simulink model "Lab2_Model"  (R2017a)
settings: Solver=VariableStepAuto  StartTime=0.0  StopTime=2  RelTol=1e-3
values from neighbouring files (symbols this model uses):
  C_D = c2d(C,0.005,'tustin')    [Lab2.m]    (also in Lab3.m = c2d(C,T,'tustin'))
  K1 = 0.66538    [Lab2.m]    (also in Lab3.m)
  Kp = 15    [Lab2.m]    (also in Lab3.m)
  p = 10.5    [Lab2.m]    (also in Lab3.m)
  T = 0.005    [Lab2.m]    (also in Lab3.m; Lab3calculations.m)
  tau = 0.030541    [Lab2.m]    (also in Lab3.m)
  z = 10    [Lab2.m]    (also in Lab3.m)
settings Model: Creator=jrampert  LastModifiedBy=jrampert

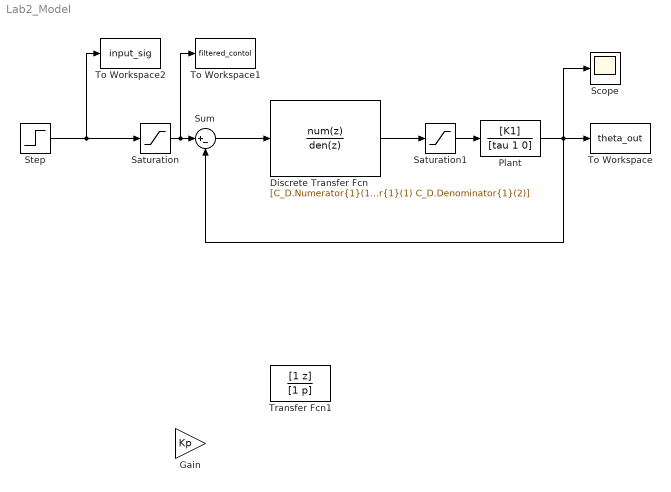
== system Lab2_Model ==
  Discrete Transfer Fcn : DiscreteTransferFcn  Numerator=[C_D.Numerator{1}(1) C_D.Numerator{1}(2)]  Denominator=[C_D.Denominator{1}(1) C_D.Denominator{1}(2)]  SampleTime=T
  Gain : Gain  Gain=Kp
  Plant : TransferFcn  Numerator=[K1]  Denominator=[tau 1 0]
  Saturation : Saturate  UpperLimit=0.785  LowerLimit=-0.785
  Saturation1 : Saturate  UpperLimit=6  LowerLimit=-6
  Scope : Scope
  Step : Step  Before=-0.7  After=0.7  SampleTime=0
  Sum : Sum  Inputs=|+-
  To Workspace : ToWorkspace  VariableName=theta_out  SaveFormat=Timeseries  SampleTime=-1
  To Workspace1 : ToWorkspace  VariableName=filtered_contol  SaveFormat=Timeseries  SampleTime=-1
  To Workspace2 : ToWorkspace  VariableName=input_sig  SaveFormat=Timeseries  SampleTime=-1
  Transfer Fcn1 : TransferFcn  Numerator=[1 z]  Denominator=[1 p]
  wires:
  Saturation/1 -> To Workspace1/1, Sum/1
  Plant/1 -> Scope/1, Sum/2, To Workspace/1
  Step/1 -> To Workspace2/1, Saturation/1
  Sum/1 -> Discrete Transfer Fcn/1
  Discrete Transfer Fcn/1 -> Saturation1/1
  Saturation1/1 -> Plant/1
